simulink model "Carrier_HeavyDelivery_UAV"  (R2025b)
settings: Solver=ode4  StartTime=0.0  StopTime=inf  FixedStep=1/60  RelTol=1e-3
libraries: dspnetwork x3, uavsim3dlib x2, sim3dlib x1
settings Model: Creator=User  LastModifiedBy=User

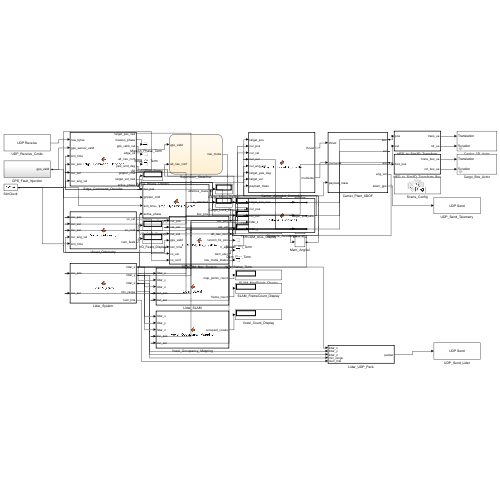
[thumbnail: Simulink's stored preview of the top-level diagram]
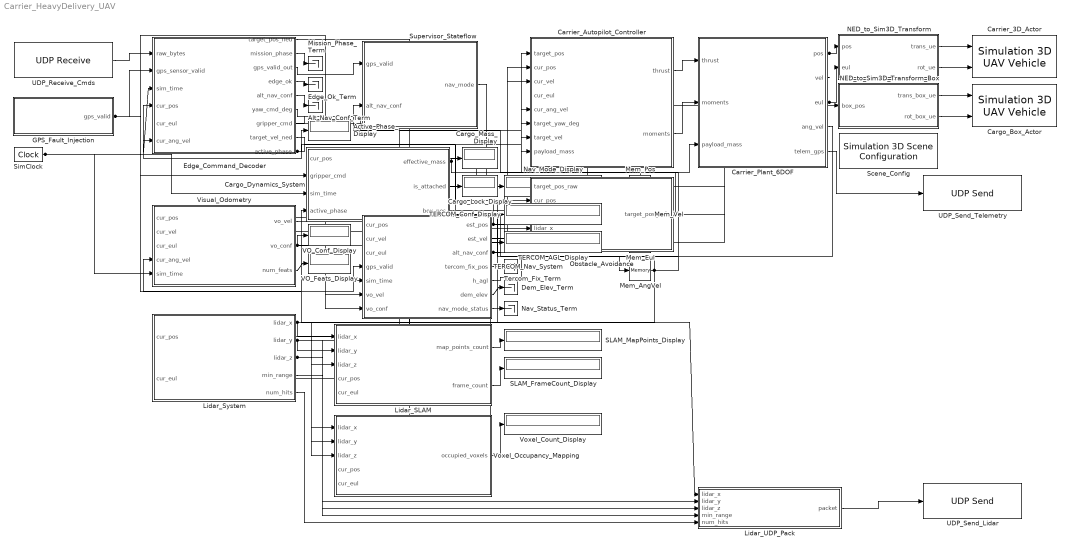
== system Carrier_HeavyDelivery_UAV ==
  Active_Phase_Display : Display
  Alt_Nav_Conf_Term : Terminator
  Cargo_Box_Actor : uavsim3dlib/Simulation 3D UAV Vehicle  Priority=-1  Mesh=Quadrotor  MeshPath=/MathWorksUAVContent/UAVs/HexaRotorUAV/HexaRotor.HexaRotor  Color=Black  ActorName=CargoBox  UseGlobalFrame=off  InitialTranslation=[0 0 0]  InitialRotation=[0 0 0]  InitialTranslationGlobal=[0 0 0]  InitialGeoOrigin=[0 0 0]  InitialRotationGlobal=[0 0 0]  SampleTime=-1  ActorType=SimulinkVehicle  ID=C  aMode=4  ActorTag=CargoBox
  Cargo_Dynamics_System : MATLAB Function  TreatAsAtomicUnit=on
  Cargo_Lock_Display : Display
  Cargo_Mass_Display : Display
  Carrier_3D_Actor : uavsim3dlib/Simulation 3D UAV Vehicle  Priority=-1  Mesh=Quadrotor  MeshPath=/MathWorksUAVContent/UAVs/HexaRotorUAV/HexaRotor.HexaRotor  Color=Black  ActorName=SimulinkVehicle1  UseGlobalFrame=off  InitialTranslation=[0 0 0]  InitialRotation=[0 0 0]  InitialTranslationGlobal=[0 0 0]  InitialGeoOrigin=[0 0 0]  InitialRotationGlobal=[0 0 0]  SampleTime=-1  ActorType=SimulinkVehicle  ID=1  aMode=4  ActorTag=SimulinkVehicle1
  Carrier_Autopilot_Controller : MATLAB Function  TreatAsAtomicUnit=on
  Carrier_Plant_6DOF : MATLAB Function  TreatAsAtomicUnit=on
  Dem_Elev_Term : Terminator
  Edge_Command_Decoder : MATLAB Function  TreatAsAtomicUnit=on
  Edge_Ok_Term : Terminator
  GPS_Fault_Injection : Subsystem
  Lidar_SLAM : MATLAB Function  TreatAsAtomicUnit=on
  Lidar_System : MATLAB Function  TreatAsAtomicUnit=on
  Lidar_UDP_Pack : MATLAB Function  TreatAsAtomicUnit=on
  Mem_AngVel : Memory  InitialCondition=[0; 0; 0]
  Mem_Eul : Memory  InitialCondition=[0; 0; 0]
  Mem_Pos : Memory  InitialCondition=[0; 0; 0]
  Mem_Vel : Memory  InitialCondition=[0; 0; 0]
  Mission_Phase_Term : Terminator
  NED_to_Sim3D_Transform : MATLAB Function  TreatAsAtomicUnit=on
  NED_to_Sim3D_Transform_Box : MATLAB Function  TreatAsAtomicUnit=on
  Nav_Mode_Display : Display
  Nav_Status_Term : Terminator
  Obstacle_Avoidance : MATLAB Function  TreatAsAtomicUnit=on
  SLAM_FrameCount_Display : Display
  SLAM_MapPoints_Display : Display
  Scene_Config : sim3dlib/Simulation 3D Scene Configuration  Priority=0  ProjectFormat=Default Scenes  SceneDesc=US city block  ProjectName=D:\MLAB\toolbox\shared\sim3d_projects\automotive_project_windows\UE\WindowsNoEditor\VehicleSimulation.exe  ScenePath=/Game/Maps/USCityBlock  EnableOpenDRIVE=off  vehTagList={'Custom';'Scene Origin'}  vehTag=Scene Origin  AttachedCameraRelativeTranslation=[0 0 0]  FreeCameraDefaultInitialTranslation=[-6, 0, 2]  AttachedCameraRelativeRotation=[0 0 0]  FreeCameraDefaultInitialRotation=[0, -15, 0]  ViewpointName=Custom  FreeCameraInitialTranslation=[0, 0, 0]  ViewpointTranslation=[0, 0, 0]  FreeCameraInitialRotation=[0, 0, 0]  ViewpointRotation=[0, 0, 0]  OpVisEn=off  Ts=1/60  EnableWindow=on  EnableRemoteAccess=off  EnableWeather=off  SunAzimuth=90  SunAltitude=40.0  EnableGeospatialSun=off  Latitude=0  Longitude=0  Date=2023-01-01  Time=10:30:00  GeoTimeZone=-5.0  SunDaylightSaving=off  wind=1  clouds=10  EnableVolumetricClouds=off  CloudCoverage=0  CloudAltitude=6  fog=0  rain=0  RaindropsEffect=off  SnowDensity=0  EnableGeospatial=off  TilesetSource=Earth terrain  UseTrueOrigin=off  OriginHeight=200  OriginLatitude=40.744652  OriginLongitude=-73.988864  MapStyle=Aerial  AdditionalAssetIDs=[]  UseAdvancedSunSky=off  SolarTime=11  TimeZone=-5  Day=21  Month=9  Year=2022  UseDaylightSavingTime=on  DSTStartDay=10  DSTStartMonth=3  DSTEndDay=3  DSTEndMonth=11  DSTSwitchHour=2  sensorTag=MainCamera1  sensorId=1  sensorName=MainCamera1  mountLoc=Origin  offsetFlag=off  tmountOffset=[0, 0, 0]  rmountOffset=[0, 0, 0]  HorizontalResolution=1280  VerticalResolution=720  HorizontalFOV=60  mountPoint=[0 0 0]  mountOrientation=[0 0 0]  aMode=4  ID=1  GeoTrigger=Inactive  ViewNameList={'Custom'}  ViewTranslationList={'[0 0 0]'}  ViewRotationList={'[0 0 0]'}
      settings: LibrarySourceBlock=uavsim3dlib/Simulation 3D Scene Configuration
  SimClock : DigitalClock  SampleTime=1/60
  Supervisor_Stateflow : Stateflow chart  TreatAsAtomicUnit=on
  TERCOM_AGL_Display : Display
  TERCOM_Conf_Display : Display
  TERCOM_Nav_System : MATLAB Function  TreatAsAtomicUnit=on
  Tercom_Fix_Term : Terminator
  UDP_Receive_Cmds : dspnetwork/UDP Receive  localURL='0.0.0.0'  localPort=5001  remoteURL='0.0.0.0'  remotePort=-1  recvBufferSize=8192  dims=255  signalDatatype=uint8  isComplex=off  isVarSize=on  showBlockingTime=off  blockingTime=0  sampletime=1/60  blockPlatform=[]
  UDP_Send_Lidar : dspnetwork/UDP Send  remoteURL='127.0.0.1'  remotePort=5003  localURL='0.0.0.0'  localPortSource=Automatically determine  localPort=2048  sendBufferSize=8192  sampletime=-1  blockPlatform=[]  separateLengthPort=0
  UDP_Send_Telemetry : dspnetwork/UDP Send  remoteURL='127.0.0.1'  remotePort=5002  localURL='0.0.0.0'  localPortSource=Automatically determine  localPort=2048  sendBufferSize=8192  sampletime=-1  blockPlatform=[]  separateLengthPort=0
  VO_Conf_Display : Display
  VO_Feats_Display : Display
  Visual_Odometry : MATLAB Function  TreatAsAtomicUnit=on
  Voxel_Count_Display : Display
  Voxel_Occupancy_Mapping : MATLAB Function  TreatAsAtomicUnit=on
  wires:
  UDP_Receive_Cmds/1 -> Edge_Command_Decoder/1(raw_bytes)
  GPS_Fault_Injection/1(gps_valid) -> Edge_Command_Decoder/2(gps_sensor_valid), TERCOM_Nav_System/4(gps_valid)
  SimClock/1 -> Edge_Command_Decoder/3(sim_time), Cargo_Dynamics_System/3(sim_time), Visual_Odometry/5(sim_time), TERCOM_Nav_System/5(sim_time)
  TERCOM_Nav_System/1(est_pos) -> Edge_Command_Decoder/4(cur_pos), Lidar_SLAM/4(cur_pos), Voxel_Occupancy_Mapping/4(cur_pos), Obstacle_Avoidance/2(cur_pos), Carrier_Autopilot_Controller/2(cur_pos)
  Mem_Eul/1 -> Edge_Command_Decoder/5(cur_eul), Visual_Odometry/3(cur_eul), TERCOM_Nav_System/3(cur_eul), Lidar_SLAM/5(cur_eul), Voxel_Occupancy_Mapping/5(cur_eul), Obstacle_Avoidance/3(cur_eul), Carrier_Autopilot_Controller/4(cur_eul), Lidar_System/2(cur_eul)
  Mem_AngVel/1 -> Edge_Command_Decoder/6(cur_ang_vel), Visual_Odometry/4(cur_ang_vel), Carrier_Autopilot_Controller/5(cur_ang_vel)
  Edge_Command_Decoder/2(mission_phase) -> Mission_Phase_Term/1
  Edge_Command_Decoder/3(gps_valid_out) -> Supervisor_Stateflow/1(gps_valid)
  Edge_Command_Decoder/4(edge_ok) -> Edge_Ok_Term/1
  Edge_Command_Decoder/5(alt_nav_conf) -> Alt_Nav_Conf_Term/1
  Edge_Command_Decoder/9(active_phase) -> Active_Phase_Display/1, Cargo_Dynamics_System/4(active_phase)
  Mem_Pos/1 -> Cargo_Dynamics_System/1(cur_pos), Visual_Odometry/1(cur_pos), TERCOM_Nav_System/1(cur_pos), Lidar_System/1(cur_pos)
  Edge_Command_Decoder/7(gripper_cmd) -> Cargo_Dynamics_System/2(gripper_cmd)
  Cargo_Dynamics_System/1(effective_mass) -> Cargo_Mass_Display/1, Carrier_Autopilot_Controller/8(payload_mass), Carrier_Plant_6DOF/3(payload_mass)
  Cargo_Dynamics_System/2(is_attached) -> Cargo_Lock_Display/1
  Supervisor_Stateflow/1(nav_mode) -> Nav_Mode_Display/1
  TERCOM_Nav_System/3(alt_nav_conf) -> Supervisor_Stateflow/2(alt_nav_conf), TERCOM_Conf_Display/1
  Mem_Vel/1 -> Visual_Odometry/2(cur_vel), TERCOM_Nav_System/2(cur_vel)
  Visual_Odometry/2(vo_conf) -> VO_Conf_Display/1, TERCOM_Nav_System/7(vo_conf)
  Visual_Odometry/3(num_feats) -> VO_Feats_Display/1
  Visual_Odometry/1(vo_vel) -> TERCOM_Nav_System/6(vo_vel)
  TERCOM_Nav_System/4(tercom_fix_pos) -> Tercom_Fix_Term/1
  TERCOM_Nav_System/5(h_agl) -> TERCOM_AGL_Display/1
  TERCOM_Nav_System/6(dem_elev) -> Dem_Elev_Term/1
  TERCOM_Nav_System/7(nav_mode_status) -> Nav_Status_Term/1
  Lidar_System/1(lidar_x) -> Lidar_SLAM/1(lidar_x), Voxel_Occupancy_Mapping/1(lidar_x), Obstacle_Avoidance/4(lidar_x), Lidar_UDP_Pack/1(lidar_x)
  Lidar_System/2(lidar_y) -> Lidar_SLAM/2(lidar_y), Voxel_Occupancy_Mapping/2(lidar_y), Obstacle_Avoidance/5(lidar_y), Lidar_UDP_Pack/2(lidar_y)
  Lidar_System/3(lidar_z) -> Lidar_SLAM/3(lidar_z), Voxel_Occupancy_Mapping/3(lidar_z), Lidar_UDP_Pack/3(lidar_z)
  Lidar_SLAM/1(map_points_count) -> SLAM_MapPoints_Display/1
  Lidar_SLAM/2(frame_count) -> SLAM_FrameCount_Display/1
  Voxel_Occupancy_Mapping/1(occupied_voxels) -> Voxel_Count_Display/1
  Edge_Command_Decoder/1(target_pos_ned) -> Obstacle_Avoidance/1(target_pos_raw)
  Obstacle_Avoidance/1(target_pos_safe) -> Carrier_Autopilot_Controller/1(target_pos)
  TERCOM_Nav_System/2(est_vel) -> Carrier_Autopilot_Controller/3(cur_vel)
  Edge_Command_Decoder/6(yaw_cmd_deg) -> Carrier_Autopilot_Controller/6(target_yaw_deg)
  Edge_Command_Decoder/8(target_vel_ned) -> Carrier_Autopilot_Controller/7(target_vel)
  Carrier_Autopilot_Controller/1(thrust) -> Carrier_Plant_6DOF/1(thrust)
  Carrier_Autopilot_Controller/2(moments) -> Carrier_Plant_6DOF/2(moments)
  Carrier_Plant_6DOF/1(pos) -> Mem_Pos/1, NED_to_Sim3D_Transform/1(pos)
  Carrier_Plant_6DOF/2(vel) -> Mem_Vel/1
  Carrier_Plant_6DOF/3(eul) -> Mem_Eul/1, NED_to_Sim3D_Transform/2(eul)
  Carrier_Plant_6DOF/4(ang_vel) -> Mem_AngVel/1
  Lidar_System/4(min_range) -> Lidar_UDP_Pack/4(min_range)
  Lidar_System/5(num_hits) -> Lidar_UDP_Pack/5(num_hits)
  Lidar_UDP_Pack/1(packet) -> UDP_Send_Lidar/1
  NED_to_Sim3D_Transform/1(trans_ue) -> Carrier_3D_Actor/1
  NED_to_Sim3D_Transform/2(rot_ue) -> Carrier_3D_Actor/2
  Cargo_Dynamics_System/3(box_pos) -> NED_to_Sim3D_Transform_Box/1(box_pos)
  NED_to_Sim3D_Transform_Box/1(trans_box_ue) -> Cargo_Box_Actor/1
  NED_to_Sim3D_Transform_Box/2(rot_box_ue) -> Cargo_Box_Actor/2
  Carrier_Plant_6DOF/5(telem_gps) -> UDP_Send_Telemetry/1

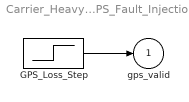
== system Carrier_HeavyDelivery_UAV/GPS_Fault_Injection ==
  GPS_Loss_Step : Step  Time=140  Before=1  After=0  SampleTime=1/60
  gps_valid : Outport
  wires:
  ? -> ?
  GPS_Loss_Step/1 -> gps_valid/1

== matlab function Carrier_HeavyDelivery_UAV/Voxel_Occupancy_Mapping ==
  data: lidar_x input; occupied_voxels output; lidar_y input; lidar_z input; cur_pos input; cur_eul input
function occupied_voxels = Voxel_Occupancy_Mapping(lidar_x, lidar_y, lidar_z, cur_pos, cur_eul)
coder.extrinsic('voxelMapUpdate');
occupied_voxels = 0.0;
occupied_voxels = voxelMapUpdate(lidar_x, lidar_y, lidar_z, cur_pos, cur_eul);

== matlab function Carrier_HeavyDelivery_UAV/Carrier_Autopilot_Controller ==
  data: target_pos input; thrust output; cur_pos input; cur_vel input; cur_eul input; cur_ang_vel input; target_yaw_deg input; target_vel input; payload_mass input; moments output
function [thrust, moments] = Carrier_Autopilot_Controller(target_pos, cur_pos, cur_vel, cur_eul, cur_ang_vel, target_yaw_deg, target_vel, payload_mass)
thrust = 0.0; moments = [0.0; 0.0; 0.0];
persistent int_vel_err int_att_err int_z_err last_vel_err
if isempty(int_vel_err)
    int_vel_err = [0.0; 0.0]; int_att_err = [0.0; 0.0; 0.0]; int_z_err = 0.0; last_vel_err = [0.0; 0.0];
end
if cur_pos(3) >= -0.10 && target_pos(3) >= -0.05
    thrust = 0.0; moments = [0.0; 0.0; 0.0];
    int_vel_err = [0.0; 0.0]; int_att_err = [0.0; 0.0; 0.0]; int_z_err = 0.0;
    return;
end
dt = 1/60; m = payload_mass; g = 9.81;
kp_v = 4.8; ki_v = 0.45; kd_v = 0.40;
e_vel = target_vel(1:2) - cur_vel(1:2);
d_vel_err = (e_vel - last_vel_err) / dt;
last_vel_err = e_vel;
e_pos = target_pos(1:2) - cur_pos(1:2);
int_vel_err = max(min(int_vel_err + (e_vel * dt), 2.5), -2.5);
acc_world = kp_v * e_vel + ki_v * int_vel_err + kd_v * d_vel_err + 0.95 * e_pos;
yaw_now = cur_eul(3);
acc_body_x =  acc_world(1) * cos(yaw_now) + acc_world(2) * sin(yaw_now);
acc_body_y = -acc_world(1) * sin(yaw_now) + acc_world(2) * cos(yaw_now);
MAX_TILT = 22 * pi / 180;
pitch_cmd = max(min(-acc_body_x / g, MAX_TILT), -MAX_TILT);
roll_cmd  = max(min( acc_body_y / g, MAX_TILT), -MAX_TILT);
kp_z = 8.5; ki_z = 1.80; kd_z = 6.0;
e_pos_z = target_pos(3) - cur_pos(3); e_vel_z = target_vel(3) - cur_vel(3);
h_agl = max(0.0, -cur_pos(3));
if h_agl < 0.8
    int_z_err = max(min(int_z_err + (e_pos_z * dt), 0.5), -0.5);
else
    int_z_err = max(min(int_z_err + (e_pos_z * dt), 3.0), -3.0);
end
thrust_raw = m * (g - kp_z * e_pos_z - ki_z * int_z_err - kd_z * e_vel_z);
cos_tilt = cos(cur_eul(1)) * cos(cur_eul(2));
thrust = max(0, min(thrust_raw / max(cos_tilt, 0.65), 2.4 * m * g));
kp_att = [24.0; 24.0; 12.0]; ki_att = [2.0; 2.0; 0.5]; kd_att = [3.5; 3.5; 2.2];
yaw_target_rad = target_yaw_deg * pi / 180;
yaw_err = atan2(sin(yaw_target_rad - cur_eul(3)), cos(yaw_target_rad - cur_eul(3)));
att_err = [roll_cmd - cur_eul(1); pitch_cmd - cur_eul(2); yaw_err];
int_att_err = max(min(int_att_err + (att_err * dt), 0.8), -0.8);
mom_calc = kp_att .* att_err + ki_att .* int_att_err - kd_att .* cur_ang_vel;
moments = [max(min(mom_calc(1), 14.0), -14.0); ...
           max(min(mom_calc(2), 14.0), -14.0); ...
           max(min(mom_calc(3), 14.0), -14.0)];

== matlab function Carrier_HeavyDelivery_UAV/Carrier_Plant_6DOF ==
  data: thrust input; pos output; moments input; payload_mass input; vel output; eul output; ang_vel output; telem_gps output
function [pos, vel, eul, ang_vel, telem_gps] = Carrier_Plant_6DOF(thrust, moments, payload_mass)
pos = [0.0; 0.0; 0.0]; vel = [0.0; 0.0; 0.0]; eul = [0.0; 0.0; 0.0]; ang_vel = [0.0; 0.0; 0.0];
telem_gps = zeros(12, 1);
persistent p v e w buildings
if isempty(p)
    p = [0; 0; 0]; v = [0; 0; 0]; e = [0; 0; 0]; w = [0; 0; 0];
    buildings = [
         8.0,  32.0, -38.0, -14.0, 45.0;
         8.0,  32.0,  18.0,  40.0, 45.0;
        36.0,  58.0,  -8.0,  16.0, 45.0;
       -32.0,  -8.0, -28.0,  -6.0, 45.0;
       -32.0,  -8.0,  10.0,  32.0, 45.0
    ];
end
dt = 1/60; m = payload_mass; g = 9.81;
if m > 16.0
    I = diag([1.28, 1.28, 0.94]); r_safe = 0.95;
else
    I = diag([0.42, 0.42, 0.78]); r_safe = 0.65;
end
phi = e(1); theta = e(2); psi = e(3);
R = [cos(theta)*cos(psi), sin(phi)*sin(theta)*cos(psi)-cos(phi)*sin(psi), cos(phi)*sin(theta)*cos(psi)+sin(phi)*sin(psi);
     cos(theta)*sin(psi), sin(phi)*sin(theta)*sin(psi)+cos(phi)*cos(psi), cos(phi)*sin(theta)*sin(psi)-sin(phi)*cos(psi);
    -sin(theta),          sin(phi)*cos(theta),                            cos(phi)*cos(theta)];
f_body = [0; 0; -thrust];
acc = (R * f_body + [0; 0; m*g]) / m;
v = v + acc * dt; p = p + v * dt;
if m > 16.0 && p(3) > -0.60
    p(3) = -0.60;
    if v(3) > 0.0; v(3) = -v(3) * 0.04; end
    v(1:2) = v(1:2) * 0.75; w = w * 0.35;
elseif p(3) > 0.0
    p(3) = 0.0;
    if v(3) > 0.0; v(3) = -v(3) * 0.05; end
    v(1:2) = v(1:2) * 0.70; w = w * 0.35;
end
drone_alt = -p(3);
for i = 1:size(buildings, 1)
    bx1 = buildings(i, 1) - r_safe; bx2 = buildings(i, 2) + r_safe;
    by1 = buildings(i, 3) - r_safe; by2 = buildings(i, 4) + r_safe;
    bh  = buildings(i, 5);
    if drone_alt <= bh && p(1) >= bx1 && p(1) <= bx2 && p(2) >= by1 && p(2) <= by2
        d_left = p(1) - bx1; d_right = bx2 - p(1);
        d_bottom = p(2) - by1; d_top = by2 - p(2);
        min_d = min([d_left, d_right, d_bottom, d_top]);
        if min_d == d_left;       p(1) = bx1; v(1) = min(v(1), 0.0);
        elseif min_d == d_right;  p(1) = bx2; v(1) = max(v(1), 0.0);
        elseif min_d == d_bottom; p(2) = by1; v(2) = min(v(2), 0.0);
        else;                     p(2) = by2; v(2) = max(v(2), 0.0);
        end
    end
end
ang_acc = I \ (moments - cross(w, I * w));
w = max(min(w + ang_acc * dt, 2.2), -2.2);
T = [1, sin(e(1))*tan(e(2)), cos(e(1))*tan(e(2)); 0, cos(e(1)), -sin(e(1)); 0, sin(e(1))/cos(e(2)), cos(e(1))/cos(e(2))];
e = e + (T * w) * dt;
pos = [p(1); p(2); p(3)]; vel = [v(1); v(2); v(3)];
eul = [e(1); e(2); e(3)]; ang_vel = [w(1); w(2); w(3)];
ref_lat = 26.99484; ref_lon = 88.28542;
lat = ref_lat + (p(1) / 111320.0);
lon = ref_lon + (p(2) / (111320.0 * cos(ref_lat * pi / 180)));
telem_gps = [lat; lon; -p(3); v(1); v(2); v(3); e(1); e(2); e(3); w(1); w(2); w(3)];

== matlab function Carrier_HeavyDelivery_UAV/Lidar_System ==
  data: cur_pos input; lidar_x output; cur_eul input; lidar_y output; lidar_z output; min_range output; num_hits output
function [lidar_x, lidar_y, lidar_z, min_range, num_hits] = Lidar_System(cur_pos, cur_eul)
N_AZ = 40; ELEVS = [-20, -10, 0, 10, 20] * pi / 180; N_EL = numel(ELEVS); N = N_AZ * N_EL;
MAX_RANGE = 30.0;
lidar_x = zeros(N, 1); lidar_y = zeros(N, 1); lidar_z = zeros(N, 1);
min_range = MAX_RANGE; num_hits = 0.0;
persistent buildings
if isempty(buildings)
    buildings = [
         8.0,  32.0, -38.0, -14.0, 45.0;
         8.0,  32.0,  18.0,  40.0, 45.0;
        36.0,  58.0,  -8.0,  16.0, 45.0;
       -32.0,  -8.0, -28.0,  -6.0, 45.0;
       -32.0,  -8.0,  10.0,  32.0, 45.0
    ];
end
phi = cur_eul(1); theta = cur_eul(2); psi = cur_eul(3);
R = [cos(theta)*cos(psi), sin(phi)*sin(theta)*cos(psi)-cos(phi)*sin(psi), cos(phi)*sin(theta)*cos(psi)+sin(phi)*sin(psi);
     cos(theta)*sin(psi), sin(phi)*sin(theta)*sin(psi)+cos(phi)*cos(psi), cos(phi)*sin(theta)*sin(psi)-sin(phi)*cos(psi);
    -sin(theta),          sin(phi)*cos(theta),                            cos(phi)*cos(theta)];
az_local = ((-pi + (0:N_AZ-1) * (2*pi/N_AZ))');
az_rep   = repmat(az_local, N_EL, 1);
el_rep   = repelem(ELEVS(:), N_AZ);
d_bx = cos(el_rep) .* cos(az_rep);
d_by = cos(el_rep) .* sin(az_rep);
d_bz = -sin(el_rep);
body_rays = [d_bx'; d_by'; d_bz'];
world_rays = R * body_rays;
ox = cur_pos(1); oy = cur_pos(2); oz = cur_pos(3);
best_t = MAX_RANGE * ones(N, 1); hit_flags = false(N, 1);
for i = 1:N
    dx = world_rays(1, i); dy = world_rays(2, i); dz = world_rays(3, i);
    if dz > 1e-4
        tg = (0.0 - oz) / dz;
        if tg > 0.0 && tg < best_t(i); best_t(i) = tg; hit_flags(i) = true; end
    end
    for b = 1:size(buildings, 1)
        bx1 = buildings(b, 1); bx2 = buildings(b, 2);
        by1 = buildings(b, 3); by2 = buildings(b, 4);
        bz1 = -buildings(b, 5); bz2 = 0.0;
        inv_x = 1.0 / (dx + sign(dx)*1e-6);
        inv_y = 1.0 / (dy + sign(dy)*1e-6);
        inv_z = 1.0 / (dz + sign(dz)*1e-6);
        tx1 = (bx1 - ox) * inv_x; tx2 = (bx2 - ox) * inv_x;
        ty1 = (by1 - oy) * inv_y; ty2 = (by2 - oy) * inv_y;
        tz1 = (bz1 - oz) * inv_z; tz2 = (bz2 - oz) * inv_z;
        tmin = max([min(tx1, tx2), min(ty1, ty2), min(tz1, tz2)]);
        tmax = min([max(tx1, tx2), max(ty1, ty2), max(tz1, tz2)]);
        if tmax >= max(tmin, 0.0) && tmin < best_t(i)
            best_t(i) = tmin; hit_flags(i) = true;
        end
    end
    if hit_flags(i)
        lidar_x(i) = best_t(i) * d_bx(i);
        lidar_y(i) = best_t(i) * d_by(i);
        lidar_z(i) = best_t(i) * d_bz(i);
    else
        lidar_x(i) = 0.0; lidar_y(i) = 0.0; lidar_z(i) = 0.0;
    end
end
num_hits = double(sum(hit_flags));
if any(hit_flags); min_range = min(best_t(hit_flags)); end
coder.extrinsic('lidarLivePlot');
midStart = 2*N_AZ + 1; midEnd = 3 * N_AZ;
lidarLivePlot(lidar_x(midStart:midEnd), lidar_y(midStart:midEnd), min_range, num_hits);

== matlab function Carrier_HeavyDelivery_UAV/Obstacle_Avoidance ==
  data: target_pos_raw input; target_pos_safe output; cur_pos input; cur_eul input; lidar_x input; lidar_y input
function target_pos_safe = Obstacle_Avoidance(target_pos_raw, cur_pos, cur_eul, lidar_x, lidar_y)
target_pos_safe = [target_pos_raw(1); target_pos_raw(2); target_pos_raw(3)];
SAFETY_RANGE = 5.5; AVOID_GAIN = 1.9;
horiz_dist = sqrt(lidar_x.^2 + lidar_y.^2);
valid = horiz_dist > 0.8 & horiz_dist < SAFETY_RANGE;
if any(valid)
    valid_ranges = horiz_dist(valid);
    [minR, idx_sub] = min(valid_ranges);
    valid_indices = find(valid);
    idx = valid_indices(idx_sub);
    yaw = cur_eul(3); c = cos(yaw); s = sin(yaw);
    wx = c * lidar_x(idx) - s * lidar_y(idx);
    wy = s * lidar_x(idx) + c * lidar_y(idx);
    push = AVOID_GAIN * (SAFETY_RANGE - minR) / SAFETY_RANGE;
    target_pos_safe(1) = target_pos_raw(1) - (wx / max(minR, 0.2)) * push * 2.0;
    target_pos_safe(2) = target_pos_raw(2) - (wy / max(minR, 0.2)) * push * 2.0;
end

== matlab function Carrier_HeavyDelivery_UAV/Lidar_UDP_Pack ==
  data: lidar_x input; packet output; lidar_y input; lidar_z input; min_range input; num_hits input
function packet = Lidar_UDP_Pack(lidar_x, lidar_y, lidar_z, min_range, num_hits)
packet = [double(numel(lidar_x)); lidar_x(:); lidar_y(:); lidar_z(:); double(min_range); double(num_hits)];

== matlab function Carrier_HeavyDelivery_UAV/NED_to_Sim3D_Transform ==
  data: pos input; trans_ue output; eul input; rot_ue output
function [trans_ue, rot_ue] = NED_to_Sim3D_Transform(pos, eul)
trans_ue = [pos(1); -pos(2); -pos(3)];
rot_ue   = [eul(1); -eul(2); -eul(3)];

== matlab function Carrier_HeavyDelivery_UAV/NED_to_Sim3D_Transform_Box ==
  data: box_pos input; trans_box_ue output; rot_box_ue output
function [trans_box_ue, rot_box_ue] = NED_to_Sim3D_Transform_Box(box_pos)
trans_box_ue = [box_pos(1); -box_pos(2); -box_pos(3)];
rot_box_ue   = [0.0; 0.0; 0.0];

== matlab function Carrier_HeavyDelivery_UAV/Cargo_Dynamics_System ==
  data: cur_pos input; effective_mass output; gripper_cmd input; sim_time input; active_phase input; is_attached output; box_pos output
function [effective_mass, is_attached, box_pos] = Cargo_Dynamics_System(cur_pos, gripper_cmd, sim_time, active_phase)
coder.extrinsic('cargoLivePlot');
effective_mass = 14.0;
is_attached = 0.0;
box_pos = [18.0; 12.0; 0.0];

persistent payload_state p_box
if isempty(payload_state)
    payload_state = 0; p_box = [18.0; 12.0; 0.0];
end

m_dry = 14.0; m_box = 6.0;

if payload_state == 0
    dist_to_box = norm(cur_pos(1:2) - p_box(1:2));
    if gripper_cmd > 0.5 && dist_to_box < 0.40 && abs(cur_pos(3) - (-0.65)) < 0.15
        payload_state = 1;
    end
elseif payload_state == 1
    if gripper_cmd < 0.5
        payload_state = 2;
        p_box = [cur_pos(1); cur_pos(2); 0.0];
    else
        p_box = [cur_pos(1); cur_pos(2); cur_pos(3) + 0.35];
    end
end

if payload_state == 1
    effective_mass = m_dry + m_box; is_attached = 1.0;
else
    effective_mass = m_dry; is_attached = 0.0;
end
box_pos = [p_box(1); p_box(2); p_box(3)];
cargoLivePlot(cur_pos, box_pos, is_attached, effective_mass, active_phase, sim_time);

== matlab function Carrier_HeavyDelivery_UAV/Edge_Command_Decoder ==
  data: raw_bytes input; target_pos_ned output; gps_sensor_valid input; sim_time input; cur_pos input; cur_eul input; cur_ang_vel input; mission_phase output; gps_valid_out output; edge_ok output; alt_nav_conf output; yaw_cmd_deg output; gripper_cmd output; target_vel_ned output; active_phase output
function [target_pos_ned, mission_phase, gps_valid_out, edge_ok, alt_nav_conf, yaw_cmd_deg, gripper_cmd, target_vel_ned, active_phase] = Edge_Command_Decoder(raw_bytes, gps_sensor_valid, sim_time, cur_pos, cur_eul, cur_ang_vel)
target_pos_ned = [0.0; 0.0; 0.0];
target_vel_ned = [0.0; 0.0; 0.0];
gps_valid_out  = double(gps_sensor_valid);
edge_ok        = 1.0;
alt_nav_conf   = 0.94;
yaw_cmd_deg    = 0.0;
gripper_cmd    = 0.0;
active_phase   = 1.0;
mission_phase  = 1.0;

persistent phase dwell_timer settled_frames
if isempty(phase)
    phase = 1; dwell_timer = 0.0; settled_frames = 0;
end

CRUISE_ALT = -15.0;
FLARE_ALT  = -2.0;
LATCH_ALT  = -0.65;
PICK_X = 18.0; PICK_Y = 12.0;
DROP_X = 45.0; DROP_Y = -20.0;
dt = 1/60;
target_mission = [0.0; 0.0; CRUISE_ALT];
v_max = 5.0; v_z_max = 1.8;

switch phase
    case 1 % Takeoff to cruise altitude
        target_mission = [0.0; 0.0; CRUISE_ALT];
        gripper_cmd = 0.0; v_max = 4.0;
        if abs(cur_pos(3) - CRUISE_ALT) < 0.6; phase = 2; end
        
    case 2 % Ingress to Pickup Zone Overhead
        target_mission = [PICK_X; PICK_Y; CRUISE_ALT];
        gripper_cmd = 0.0; v_max = 5.0;
        if norm(cur_pos(1:2) - [PICK_X; PICK_Y]) < 0.6; phase = 3; end
        
    case 3 % Flared Approach to Pre-Contact Holding Point
        target_mission = [PICK_X; PICK_Y; FLARE_ALT];
        gripper_cmd = 0.0; v_max = 2.0; v_z_max = 1.2;
        if norm(cur_pos(1:2) - [PICK_X; PICK_Y]) < 0.25 && abs(cur_pos(3) - FLARE_ALT) < 0.20
            phase = 4; settled_frames = 0;
        end
        
    case 4 % Precision Creep Descent to Box Latch Plane
        target_mission = [PICK_X; PICK_Y; LATCH_ALT];
        gripper_cmd = 0.0; v_max = 0.40; v_z_max = 0.22;
        d_xy = norm(cur_pos(1:2) - [PICK_X; PICK_Y]);
        d_z  = abs(cur_pos(3) - LATCH_ALT);
        if d_xy < 0.15 && d_z < 0.05; settled_frames = settled_frames + 1;
        else; settled_frames = 0; end
        if settled_frames > 20; phase = 5; dwell_timer = 0.0; end
        
    case 5 % Gripper Latch Activation (2.0s dwell)
        target_mission = [PICK_X; PICK_Y; LATCH_ALT];
        gripper_cmd = 1.0; v_max = 0.1; v_z_max = 0.1;
        dwell_timer = dwell_timer + dt;
        if dwell_timer >= 2.0; phase = 6; end
        
    case 6 % Heavy-Laden Flared Climb
        target_mission = [PICK_X; PICK_Y; FLARE_ALT];
        gripper_cmd = 1.0; v_max = 1.5; v_z_max = 1.0;
        if abs(cur_pos(3) - FLARE_ALT) < 0.3; phase = 7; end
        
    case 7 % Heavy-Laden Climb to Cruise
        target_mission = [PICK_X; PICK_Y; CRUISE_ALT];
        gripper_cmd = 1.0; v_max = 3.0; v_z_max = 1.5;
        if abs(cur_pos(3) - CRUISE_ALT) < 0.8; phase = 8; end
        
    case 8 % Heavy Laden Cruise Transit to Dropoff Pad
        target_mission = [DROP_X; DROP_Y; CRUISE_ALT];
        gripper_cmd = 1.0; v_max = 4.2; v_z_max = 1.5;
        if norm(cur_pos(1:2) - [DROP_X; DROP_Y]) < 0.6; phase = 9; end
        
    case 9 % Flared Approach to Pre-Drop Holding Point
        target_mission = [DROP_X; DROP_Y; FLARE_ALT];
        gripper_cmd = 1.0; v_max = 2.0; v_z_max = 1.2;
        if norm(cur_pos(1:2) - [DROP_X; DROP_Y]) < 0.25 && abs(cur_pos(3) - FLARE_ALT) < 0.20
            phase = 10; settled_frames = 0;
        end
        
    case 10 % Precision Creep Descent to Delivery Surface
        target_mission = [DROP_X; DROP_Y; LATCH_ALT];
        gripper_cmd = 1.0; v_max = 0.40; v_z_max = 0.22;
        d_xy = norm(cur_pos(1:2) - [DROP_X; DROP_Y]);
        d_z  = abs(cur_pos(3) - LATCH_ALT);
        if d_xy < 0.15 && d_z < 0.05; settled_frames = settled_frames + 1;
        else; settled_frames = 0; end
        if settled_frames > 20; phase = 11; dwell_timer = 0.0; end
        
    case 11 % Release Cargo Box (2.0s dwell)
        target_mission = [DROP_X; DROP_Y; LATCH_ALT];
        gripper_cmd = 0.0; v_max = 0.1; v_z_max = 0.1;
        dwell_timer = dwell_timer + dt;
        if dwell_timer >= 2.0; phase = 12; end
        
    case 12 % Unladen Egress Climb to Cruise
        target_mission = [DROP_X; DROP_Y; CRUISE_ALT];
        gripper_cmd = 0.0; v_max = 3.5; v_z_max = 1.8;
        if abs(cur_pos(3) - CRUISE_ALT) < 0.8; phase = 13; end
        
    case 13 % High-Speed Return to Base (RTB)
        target_mission = [0.0; 0.0; CRUISE_ALT];
        gripper_cmd = 0.0; v_max = 5.0; v_z_max = 1.8;
        if norm(cur_pos(1:2) - [0.0; 0.0]) < 0.6; phase = 14; end
        
    case 14 % Final Soft Touchdown Landing
        target_mission = [0.0; 0.0; 0.0];
        gripper_cmd = 0.0; v_max = 1.0; v_z_max = 0.50;
        
    otherwise
        target_mission = [0.0; 0.0; 0.0]; gripper_cmd = 0.0;
end

active_phase = double(phase); mission_phase = double(phase);
target_pos_ned = [target_mission(1); target_mission(2); target_mission(3)];

delta_pos = target_mission - cur_pos;
dist_xy = norm(delta_pos(1:2));
v_des_xy = v_max * tanh(dist_xy / 1.5);
if dist_xy > 0.04; v_cmd_xy = v_des_xy * (delta_pos(1:2) / dist_xy);
else; v_cmd_xy = [0.0; 0.0]; end
delta_z = delta_pos(3);
v_cmd_z = sign(delta_z) * v_z_max * tanh(abs(delta_z) / 1.0);
target_vel_ned = [v_cmd_xy(1); v_cmd_xy(2); v_cmd_z];

== stateflow chart Carrier_HeavyDelivery_UAV/Supervisor_Stateflow ==
  state GPS_PRIMARY
    entry: nav_mode = 0;
  state TERCOM_ALT_NAV
    entry: nav_mode = 1;
  state INERTIAL_HOLD
    entry: nav_mode = 2;
  (default) -> GPS_PRIMARY
  INERTIAL_HOLD -> GPS_PRIMARY : [gps_valid >= 0.5]
  TERCOM_ALT_NAV -> GPS_PRIMARY [order 1] : [gps_valid >= 0.5]
  GPS_PRIMARY -> TERCOM_ALT_NAV [order 1] : [gps_valid < 0.5 && alt_nav_conf >= 0.6]
  GPS_PRIMARY -> INERTIAL_HOLD [order 2] : [gps_valid < 0.5 && alt_nav_conf < 0.6]
  TERCOM_ALT_NAV -> INERTIAL_HOLD [order 2] : [alt_nav_conf < 0.6]
  data: gps_valid input double; alt_nav_conf input double; nav_mode output double

== matlab function Carrier_HeavyDelivery_UAV/Visual_Odometry ==
  data: cur_pos input; vo_vel output; cur_vel input; cur_eul input; cur_ang_vel input; sim_time input; vo_conf output; num_feats output
function [vo_vel, vo_conf, num_feats] = Visual_Odometry(cur_pos, cur_vel, cur_eul, cur_ang_vel, sim_time)
coder.extrinsic('voLivePlot');
vo_vel = [0.0; 0.0; 0.0]; vo_conf = 0.10; num_feats = 0.0;
h_agl = max(0.0, -cur_pos(3)); N_FEATS = 32;
persistent feat_x feat_y feat_init;
if isempty(feat_init)
    feat_init = true; rng(42);
    feat_x = 1.4 * (rand(N_FEATS, 1) - 0.5);
    feat_y = 1.4 * (rand(N_FEATS, 1) - 0.5);
end
flow_u = zeros(N_FEATS, 1); flow_v = zeros(N_FEATS, 1);
if h_agl >= 0.40
    w_b = cur_ang_vel;
    R_pitch_cant = [cos(-15*pi/180), 0, sin(-15*pi/180); 0, 1, 0; -sin(-15*pi/180), 0, cos(-15*pi/180)];
    w_c = R_pitch_cant * w_b;
    Z_depth = max(0.8, h_agl);
    v_cam_truth = R_pitch_cant * cur_vel;
    for i = 1:N_FEATS
        u = feat_x(i); v = feat_y(i);
        flow_u(i) = (v_cam_truth(1) - u * v_cam_truth(3)) / Z_depth - (u*v*w_c(1) - (1 + u^2)*w_c(2) + v*w_c(3));
        flow_v(i) = (v_cam_truth(2) - v * v_cam_truth(3)) / Z_depth - ((1 + v^2)*w_c(1) - u*v*w_c(2) - u*w_c(3));
    end
    derot_u = flow_u + (feat_x.*feat_y.*w_c(1) - (1 + feat_x.^2).*w_c(2) + feat_y.*w_c(3));
    derot_v = flow_v + ((1 + feat_y.^2).*w_c(1) - feat_x.*feat_y.*w_c(2) - feat_x.*w_c(3));
    vo_vel = R_pitch_cant' * [mean(derot_u) * Z_depth; mean(derot_v) * Z_depth; cur_vel(3)];
    vo_conf = 0.90; num_feats = double(N_FEATS);
end
voLivePlot(flow_u, flow_v, feat_x, feat_y, vo_vel, vo_conf, num_feats);

== matlab function Carrier_HeavyDelivery_UAV/TERCOM_Nav_System ==
  data: cur_pos input; est_pos output; cur_vel input; cur_eul input; gps_valid input; sim_time input; vo_vel input; vo_conf input; est_vel output; alt_nav_conf output; tercom_fix_pos output; h_agl output; dem_elev output; nav_mode_status output
function [est_pos, est_vel, alt_nav_conf, tercom_fix_pos, h_agl, dem_elev, nav_mode_status] = TERCOM_Nav_System(cur_pos, cur_vel, cur_eul, gps_valid, sim_time, vo_vel, vo_conf)
est_pos = [0.0; 0.0; 0.0]; est_vel = [0.0; 0.0; 0.0];
alt_nav_conf = 0.85; tercom_fix_pos = [0.0; 0.0; 0.0];
h_agl = 0.0; dem_elev = 0.0; nav_mode_status = 0.0;
persistent p_nom v_nom R_nom ba_nom bg_nom P_cov last_time last_vel_truth fix_pos last_conf p_dr
if isempty(P_cov)
    p_nom = [0; 0; 0]; v_nom = [0; 0; 0]; R_nom = eye(3);
    ba_nom = [0.08; -0.06; 0.02]; bg_nom = [0.005; -0.004; 0.002]; p_dr = [0; 0; 0];
    P_cov = blkdiag(0.2*eye(3), 0.05*eye(3), 0.01*eye(3), 0.05*eye(3), 0.001*eye(3));
    last_time = sim_time; last_vel_truth = cur_vel; fix_pos = cur_pos; last_conf = 0.85;
end
dt = sim_time - last_time;
if dt <= 0.0 || dt > 0.1; dt = 1/60; end
last_time = sim_time;
z_dem_true = 7.5 * sin(cur_pos(1)/28.0) * cos(cur_pos(2)/24.0) + 4.0 * cos((cur_pos(1) + cur_pos(2))/20.0) + 2.5 * sin(cur_pos(2)/14.0) - 4.0;
dem_elev = z_dem_true;
true_agl = max(0.0, (-cur_pos(3)) - z_dem_true);
h_agl = true_agl + 0.04 * sin(sim_time * 12.0);
h_baro = (-cur_pos(3)) + 0.03 * cos(sim_time * 8.0);
a_truth = (cur_vel - last_vel_truth) / dt;
last_vel_truth = cur_vel;
f_spec_world = a_truth - [0; 0; 9.81];
phi = cur_eul(1); theta = cur_eul(2); psi = cur_eul(3);
R_truth = [cos(theta)*cos(psi), sin(phi)*sin(theta)*cos(psi)-cos(phi)*sin(psi), cos(phi)*sin(theta)*cos(psi)+sin(phi)*sin(psi);
           cos(theta)*sin(psi), sin(phi)*sin(theta)*sin(psi)+cos(phi)*cos(psi), cos(phi)*sin(theta)*sin(psi)-sin(phi)*cos(psi);
          -sin(theta),          sin(phi)*cos(theta),                            cos(phi)*cos(theta)];
f_b_meas = R_truth' * f_spec_world + ba_nom + 0.03 * [sin(sim_time*30); cos(sim_time*25); sin(sim_time*20)];
w_b_meas = [0; 0; 0] + bg_nom + 0.002 * [cos(sim_time*15); sin(sim_time*15); cos(sim_time*10)];
p_dr = p_dr + (cur_vel + [0.15; -0.12; 0.0]) * dt;
f_b_corr = f_b_meas - ba_nom; w_b_corr = w_b_meas - bg_nom;
w_skew = [0, -w_b_corr(3), w_b_corr(2); w_b_corr(3), 0, -w_b_corr(1); -w_b_corr(2), w_b_corr(1), 0];
R_nom = R_nom * (eye(3) + w_skew * dt);
a_nom_world = R_nom * f_b_corr + [0; 0; 9.81];
p_nom = p_nom + v_nom * dt + 0.5 * a_nom_world * (dt^2);
v_nom = v_nom + a_nom_world * dt;
if p_nom(3) > 0.0; p_nom(3) = 0.0; v_nom(3) = 0.0; end
f_skew = [0, -f_b_corr(3), f_b_corr(2); f_b_corr(3), 0, -f_b_corr(1); -f_b_corr(2), f_b_corr(1), 0];
F = eye(15); F(1:3, 4:6) = eye(3)*dt; F(4:6, 7:9) = -R_nom*f_skew*dt; F(4:6, 10:12) = -R_nom*dt; F(7:9, 7:9) = eye(3)-w_skew*dt; F(7:9, 13:15) = -eye(3)*dt;
Q = blkdiag(1e-4*eye(3), 0.02*eye(3), 1e-4*eye(3), 1e-5*eye(3), 1e-6*eye(3)) * dt;
P_cov = F * P_cov * F' + Q;
if gps_valid >= 0.5
    z_gps = [cur_pos; cur_vel]; H_gps = [eye(6), zeros(6, 9)]; R_gps = blkdiag(0.2*eye(3), 0.05*eye(3));
    y_gps = z_gps - [p_nom; v_nom]; S_gps = H_gps * P_cov * H_gps' + R_gps; K_gps = P_cov * H_gps' / S_gps;
    dx_gps = K_gps * y_gps;
    p_nom = p_nom + dx_gps(1:3); v_nom = v_nom + dx_gps(4:6);
    dth = dx_gps(7:9); dth_skew = [0, -dth(3), dth(2); dth(3), 0, -dth(1); -dth(2), dth(1), 0];
    R_nom = R_nom * (eye(3) + dth_skew);
    ba_nom = ba_nom + dx_gps(10:12); bg_nom = bg_nom + dx_gps(13:15);
    P_cov = (eye(15) - K_gps * H_gps) * P_cov;
    fix_pos = p_nom; last_conf = 0.94; nav_mode_status = 0.0;
else
    if vo_conf >= 0.35
        H_vo = [zeros(3,3), eye(3), zeros(3,9)]; R_vo = diag([0.08, 0.08, 0.12]) / max(vo_conf, 0.1);
        y_vo = vo_vel - v_nom; S_vo = H_vo * P_cov * H_vo' + R_vo; K_vo = P_cov * H_vo' / S_vo;
        dx_vo = K_vo * y_vo;
        p_nom = p_nom + dx_vo(1:3); v_nom = v_nom + dx_vo(4:6);
        P_cov = (eye(15) - K_vo * H_vo) * P_cov;
    end
    fix_pos = p_nom; last_conf = 0.88; nav_mode_status = 1.0;
end
pos_std = sqrt(max(P_cov(1,1), P_cov(2,2)));
search_win = max(6.0, min(24.0, 3.0 * pos_std));
alt_nav_conf = last_conf; tercom_fix_pos = fix_pos;
est_pos = [p_nom(1); p_nom(2); p_nom(3)];
est_vel = [v_nom(1); v_nom(2); v_nom(3)];
coder.extrinsic('tercomLivePlot');
tercomLivePlot(cur_pos, p_dr, est_pos, fix_pos, alt_nav_conf, nav_mode_status, h_baro, h_agl, dem_elev, search_win, pos_std);

== matlab function Carrier_HeavyDelivery_UAV/Lidar_SLAM ==
  data: lidar_x input; map_points_count output; lidar_y input; lidar_z input; cur_pos input; cur_eul input; frame_count output
function [map_points_count, frame_count] = Lidar_SLAM(lidar_x, lidar_y, lidar_z, cur_pos, cur_eul)
coder.extrinsic('lidarSlamUpdate');
map_points_count = 0.0;
frame_count = 0.0;
[map_points_count, frame_count] = lidarSlamUpdate(lidar_x, lidar_y, lidar_z, cur_pos, cur_eul);
